simulink model "model_nonlinear_bike_open_loop"  (R2018b)
settings: Solver=VariableStepAuto  StartTime=0.0  StopTime=60  RelTol=1e-3
values from neighbouring files (symbols this model uses):
  bike =     [bike.mat]    (also in modelconfig.mat)
  parameters =     [modelconfig.mat]
  state_space =     [modelconfig.mat]
settings Model: Creator=micha  LastModifiedBy=micha

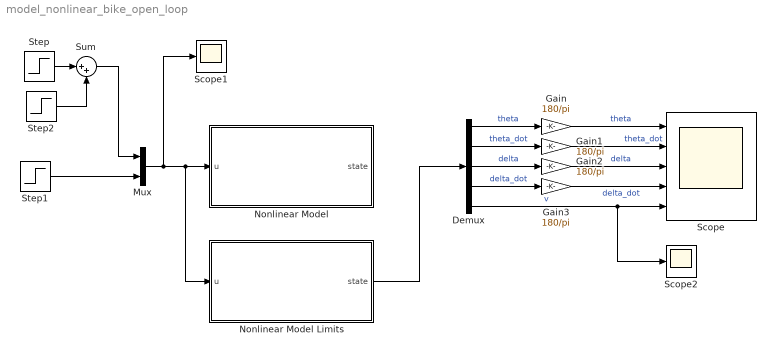
== system model_nonlinear_bike_open_loop ==
  Demux : Demux  Outputs=5
  Gain{,1..3} (4 alike) : Gain  Gain=180/pi
  Mux : Mux  Inputs=2
  Nonlinear Model : Subsystem
  Nonlinear Model Limits : Subsystem
  Scope : Scope  NumInputPorts=5
  Scope1 : Scope
  Scope2 : Scope
  Step : Step  Time=3  After=0.01  SampleTime=0
  Step1 : Step  Time=2  Before=5  After=0  SampleTime=0
  Step2 : Step  Time=4  After=-0.01  SampleTime=0
  Sum : Sum  Inputs=|++
  wires:
  Demux/1 -> Gain/1  "theta"
  Demux/2 -> Gain1/1  "theta_dot"
  Demux/3 -> Gain2/1  "delta"
  Demux/4 -> Gain3/1  "delta_dot"
  Demux/5 -> Scope2/1, Scope/5  "v"
  Step1/1 -> Mux/2
  Mux/1 -> Scope1/1, Nonlinear Model Limits/1(u), Nonlinear Model/1(u)
  Step/1 -> Sum/1
  Step2/1 -> Sum/2
  Sum/1 -> Mux/1
  Nonlinear Model Limits/1(state) -> Demux/1
  Gain/1 -> Scope/1  "theta"
  Gain1/1 -> Scope/2  "theta_dot"
  Gain2/1 -> Scope/3  "delta"
  Gain3/1 -> Scope/4  "delta_dot"

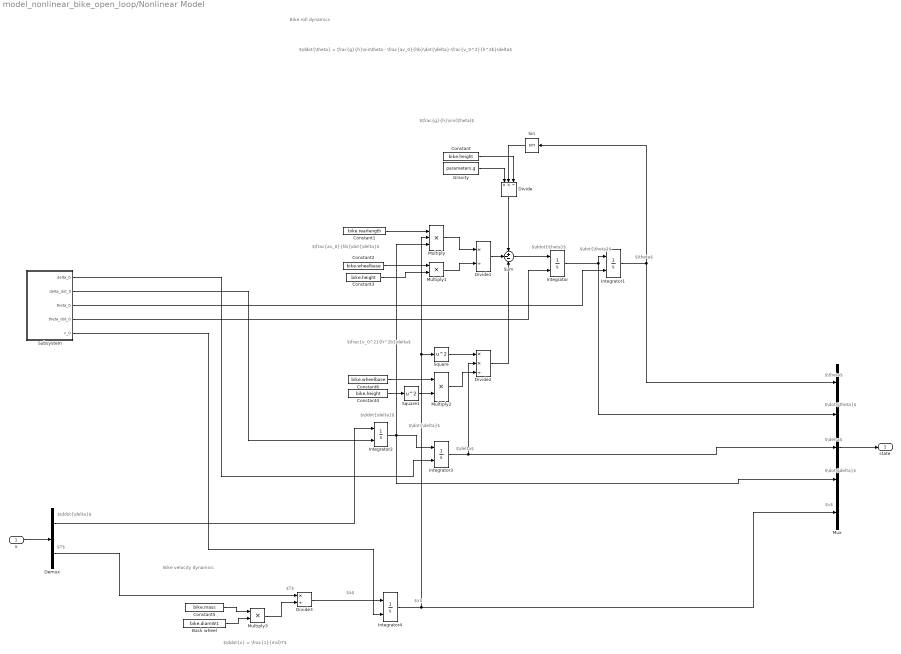
== system model_nonlinear_bike_open_loop/Nonlinear Model ==
  note: Bike velocity dynamics
  note: $\ddot{\theta} = \frac{g}{h}\sin\theta - \frac{av_0}{hb}\dot{\delta}-\frac{v_0^2}{h^2b}\delta$
  note: Bike roll dynamics
  note: $\ddot{x} = \frac{1}{md}T$
  note: $T$
  note: $v$
  note: $a$
  note: $\frac{v_0^2}{h^2b}\delta$
  note: $\frac{g}{h}\sin(\theta)$
  note: $\frac{av_0}{hb}\dot{\delta}$
  note: $\delta$
  note: $\dot{\delta}$
  note: $\ddot{\delta}$
  note: $\theta$
  note: $\dot{\theta}$
  note: $\ddot{\theta}$
  note: $\theta$
  note: $\dot{\theta}$
  note: $\delta$
  note: $\dot{\delta}$
  note: $v$
  note: $\ddot{\delta}$
  note: $T$
  u : Inport
  Back wheel : Constant  Value=bike.diamW1
  Constant : Constant  Value=bike.height
  Constant1 : Constant  Value=bike.rearlength
  Constant2 : Constant  Value=bike.wheelbase
  Constant3 : Constant  Value=bike.height
  Constant4 : Constant  Value=bike.height
  Constant5 : Constant  Value=bike.mass
  Constant6 : Constant  Value=bike.wheelbase
  Demux : Demux  Outputs=2
  Divide : Product  Inputs=**/
  Divide1 : Product  Inputs=*/
  Divide2 : Product  Inputs=**/
  Divide3 : Product  Inputs=*/
  Gravity : Constant  Value=parameters.g
  Integrator{,1..4} (5 alike) : Integrator  InitialConditionSource=external
  Multiply : Product  Inputs=3
  Multiply1 : Product
  Multiply2 : Product
  Multiply3 : Product
  Mux : Mux  Inputs=5
  Sin : Trigonometry
  Square : Math  Operator=square  SaturateOnIntegerOverflow=on
  Square1 : Math  Operator=square  SaturateOnIntegerOverflow=on
  Subsystem : Subsystem
  Sum : Sum  Inputs=+--
  state : Outport
  wires:
  Integrator/1 -> Integrator1/1, Mux/2
  Integrator1/1 -> Mux/1, Sin/1
  Sum/1 -> Integrator/1
  Divide/1 -> Sum/1
  Gravity/1 -> Divide/1
  Sin/1 -> Divide/2
  Constant/1 -> Divide/3
  Demux/1 -> Integrator2/1
  Integrator2/1 -> Integrator3/1, Mux/4, Multiply/3
  Integrator3/1 -> Mux/3, Divide2/2
  Divide1/1 -> Sum/2
  Multiply/1 -> Divide1/1
  Multiply1/1 -> Divide1/2
  Constant1/1 -> Multiply/1
  Constant2/1 -> Multiply1/1
  Constant3/1 -> Multiply1/2
  Divide2/1 -> Sum/3
  Multiply2/1 -> Divide2/3
  Constant4/1 -> Square1/1
  Constant6/1 -> Multiply2/1
  Mux/1 -> state/1
  u/1 -> Demux/1
  Integrator4/1 -> Multiply/2, Square/1, Mux/5
  Square/1 -> Divide2/1
  Square1/1 -> Multiply2/2
  Demux/2 -> Divide3/1
  Multiply3/1 -> Divide3/2
  Constant5/1 -> Multiply3/1
  Back wheel/1 -> Multiply3/2
  Divide3/1 -> Integrator4/1
  Subsystem/3(theta_0) -> Integrator1/2
  Subsystem/4(theta_dot_0) -> Integrator/2
  Subsystem/2(delta_dot_0) -> Integrator2/2
  Subsystem/1(delta_0) -> Integrator3/2
  Subsystem/5(v_0) -> Integrator4/2

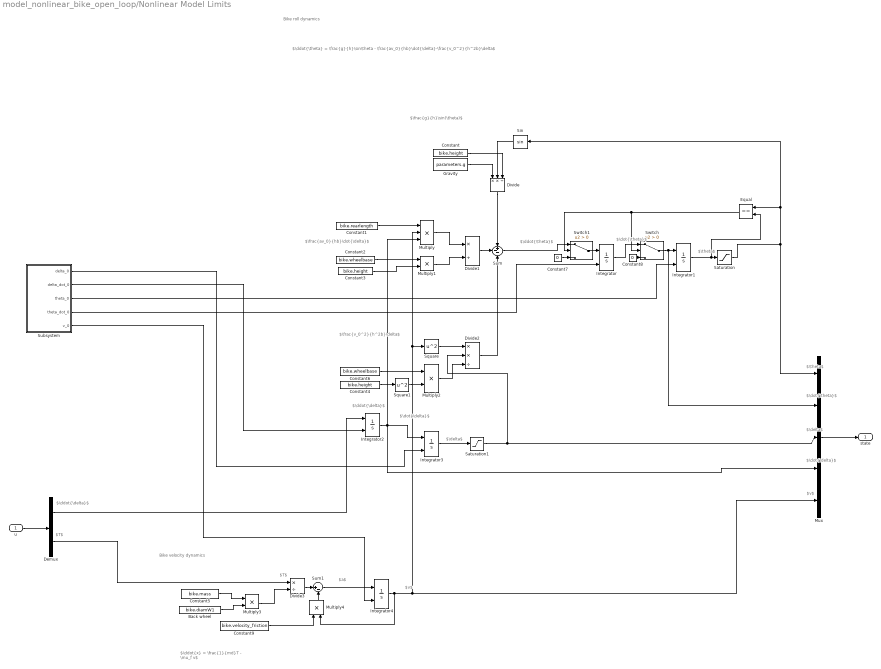
== system model_nonlinear_bike_open_loop/Nonlinear Model Limits ==
  note: Bike velocity dynamics
  note: $\ddot{\theta} = \frac{g}{h}\sin\theta - \frac{av_0}{hb}\dot{\delta}-\frac{v_0^2}{h^2b}\delta$
  note: Bike roll dynamics
  note: $\ddot{x} = \frac{1}{md}T - \mu_f v$
  note: $T$
  note: $v$
  note: $a$
  note: $\frac{v_0^2}{h^2b}\delta$
  note: $\frac{g}{h}\sin(\theta)$
  note: $\frac{av_0}{hb}\dot{\delta}$
  note: $\delta$
  note: $\dot{\delta}$
  note: $\ddot{\delta}$
  note: $\theta$
  note: $\dot{\theta}$
  note: $\ddot{\theta}$
  note: $\theta$
  note: $\dot{\theta}$
  note: $\delta$
  note: $\dot{\delta}$
  note: $v$
  note: $\ddot{\delta}$
  note: $T$
  u : Inport
  Back wheel : Constant  Value=bike.diamW1
  Constant : Constant  Value=bike.height
  Constant1 : Constant  Value=bike.rearlength
  Constant2 : Constant  Value=bike.wheelbase
  Constant3 : Constant  Value=bike.height
  Constant4 : Constant  Value=bike.height
  Constant5 : Constant  Value=bike.mass
  Constant6 : Constant  Value=bike.wheelbase
  Constant7 : Constant  Value=0
  Constant8 : Constant  Value=0
  Constant9 : Constant  Value=bike.velocity_friction
  Demux : Demux  Outputs=2
  Divide : Product  Inputs=**/
  Divide1 : Product  Inputs=*/
  Divide2 : Product  Inputs=**/
  Divide3 : Product  Inputs=*/
  Equal : RelationalOperator  Operator===  OutDataTypeStr=boolean  RndMeth=Simplest
  Gravity : Constant  Value=parameters.g
  Integrator{,1..4} (5 alike) : Integrator  InitialConditionSource=external
  Multiply : Product  Inputs=3
  Multiply{1..4} (4 alike) : Product
  Mux : Mux  Inputs=5
  Saturation : Saturate  UpperLimit=pi/2  LowerLimit=-pi/2
  Saturation1 : Saturate  UpperLimit=pi/4  LowerLimit=-pi/4
  Sin : Trigonometry
  Square : Math  Operator=square  SaturateOnIntegerOverflow=on
  Square1 : Math  Operator=square  SaturateOnIntegerOverflow=on
  Subsystem : Subsystem
  Sum : Sum  Inputs=+--
  Sum1 : Sum  Inputs=|+-
  Switch : Switch  Criteria=u2 > Threshold
  Switch1 : Switch  Criteria=u2 > Threshold
  state : Outport
  wires:
  Integrator/1 -> Switch/1
  Integrator1/1 -> Equal/2, Saturation/1
  Sum/1 -> Switch1/1
  Divide/1 -> Sum/1
  Gravity/1 -> Divide/1
  Sin/1 -> Divide/2
  Constant/1 -> Divide/3
  Demux/1 -> Integrator2/1
  Integrator2/1 -> Integrator3/1, Mux/4, Multiply/3
  Divide1/1 -> Sum/2
  Multiply/1 -> Divide1/1
  Multiply1/1 -> Divide1/2
  Constant1/1 -> Multiply/1
  Constant2/1 -> Multiply1/1
  Constant3/1 -> Multiply1/2
  Divide2/1 -> Sum/3
  Multiply2/1 -> Divide2/3
  Constant4/1 -> Square1/1
  Constant6/1 -> Multiply2/1
  Mux/1 -> state/1
  u/1 -> Demux/1
  Integrator4/1 -> Multiply/2, Square/1, Mux/5, Multiply4/2
  Square/1 -> Divide2/1
  Square1/1 -> Multiply2/2
  Demux/2 -> Divide3/1
  Multiply3/1 -> Divide3/2
  Constant5/1 -> Multiply3/1
  Back wheel/1 -> Multiply3/2
  Divide3/1 -> Sum1/1
  Subsystem/3(theta_0) -> Integrator1/2
  Subsystem/4(theta_dot_0) -> Integrator/2
  Subsystem/2(delta_dot_0) -> Integrator2/2
  Subsystem/1(delta_0) -> Integrator3/2
  Subsystem/5(v_0) -> Integrator4/2
  Saturation/1 -> Sin/1, Equal/1, Mux/1
  Integrator3/1 -> Saturation1/1
  Saturation1/1 -> Divide2/2, Mux/3
  Equal/1 -> Switch/2, Switch1/2
  Constant7/1 -> Switch1/3
  Switch/1 -> Mux/2, Integrator1/1
  Switch1/1 -> Integrator/1
  Constant8/1 -> Switch/3
  Sum1/1 -> Integrator4/1
  Multiply4/1 -> Sum1/2
  Constant9/1 -> Multiply4/1

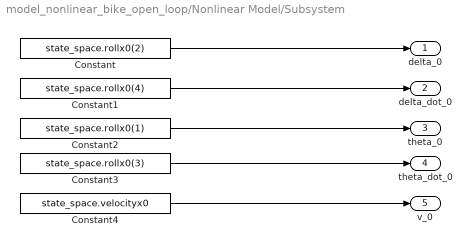
== system model_nonlinear_bike_open_loop/Nonlinear Model/Subsystem ==
  Constant : Constant  Value=state_space.rollx0(2)
  Constant1 : Constant  Value=state_space.rollx0(4)
  Constant2 : Constant  Value=state_space.rollx0(1)
  Constant3 : Constant  Value=state_space.rollx0(3)
  Constant4 : Constant  Value=state_space.velocityx0  VectorParams1D=off
  delta_0 : Outport
  delta_dot_0 : Outport  Port=2
  theta_0 : Outport  Port=3
  theta_dot_0 : Outport  Port=4
  v_0 : Outport  Port=5
  wires:
  Constant/1 -> delta_0/1
  Constant1/1 -> delta_dot_0/1
  Constant2/1 -> theta_0/1
  Constant3/1 -> theta_dot_0/1
  Constant4/1 -> v_0/1

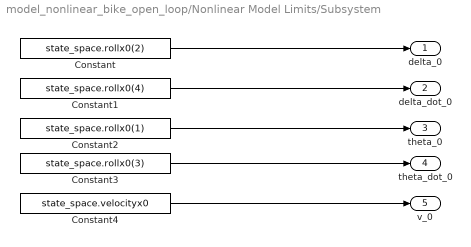
== system model_nonlinear_bike_open_loop/Nonlinear Model Limits/Subsystem ==
  Constant : Constant  Value=state_space.rollx0(2)
  Constant1 : Constant  Value=state_space.rollx0(4)
  Constant2 : Constant  Value=state_space.rollx0(1)
  Constant3 : Constant  Value=state_space.rollx0(3)
  Constant4 : Constant  Value=state_space.velocityx0  VectorParams1D=off
  delta_0 : Outport
  delta_dot_0 : Outport  Port=2
  theta_0 : Outport  Port=3
  theta_dot_0 : Outport  Port=4
  v_0 : Outport  Port=5
  wires:
  Constant/1 -> delta_0/1
  Constant1/1 -> delta_dot_0/1
  Constant2/1 -> theta_0/1
  Constant3/1 -> theta_dot_0/1
  Constant4/1 -> v_0/1
